simulink model "sample_system"  (R2022a)
settings: Solver=VariableStepAuto  StartTime=0  StopTime=t_sim_stop  RelTol=1e-3
values from neighbouring files (symbols this model uses):
  A = (pi/4)*(d_inj*.0254)^2    (= 1.14009182797e-05)    [Run_sim.m]
  attack_final_deviations = zeros(n_meas,1)    [Plot_attack_performance.m]    (also in Run_sim.m; find_non_trip_attack.m; get_simulation_object_sample_system.m; mymodelLoss.m)
  attack_full_times = attack_start_times +  100    [Plot_attack_performance.m]    (also in Run_sim.m = attack_start_times + 100; find_non_trip_attack.m; get_simulation_object_sample_system.m = attack_start_times +  10; mymodelLoss.m = attack_start_times +  10)
  attack_start_times = attack_start_injection*ones(n_meas,1)    [Plot_attack_performance.m]    (also in Run_sim.m; find_non_trip_attack.m; get_simulation_object_sample_system.m = 2*ones(n_meas,1); mymodelLoss.m = 2*ones(n_meas,1))
  Cd = 0.001    [Run_sim.m]
  detection_start = 100    [Run_sim.m]
  eta = 0.1    [Run_sim.m]
  Kd = 20    [Run_sim.m]
  Ki = 20    [Run_sim.m]
  Kp = 50    [Run_sim.m]
  noise_seed = 23341    [Run_sim.m]
  P_in = 101325    [Run_sim.m]
  P_middle = 1.68*P_in    (= 170226)    [Run_sim.m]
  P_out = 2*1.68*P_in    (= 340452)    [Run_sim.m]
  q_ref = 10    [Run_sim.m]
  x0 = [0;0]    [Run_sim.m]
libraries: slpidlib x2
settings Model: SimulationMode=rapid-accelerator  Creator=Abelb  LastModifiedBy=Abelb
settings DataIOCC: SaveFormat=StructureWithTime
settings OptimizationCC: BlockReduction=off  BufferReuse=off
settings DebuggingCC: AlgebraicLoopMsg=none
settings HardwareCC: TargetBitPerPointer=64  TargetBitPerSizeT=64  TargetBitPerPtrDiffT=64  TargetLongLongMode=on  TargetIntDivRoundTo=Zero  TargetEndianess=LittleEndian  TargetWordSize=64  TargetHWDeviceType=MATLAB Host  ProdEqTarget=off
settings RTWCC: Description=Rapid Simulation Target  SystemTargetFile=rsim.tlc  TemplateMakefile=rsim_default_tmf  DLArmComputeVersion=19.05
settings RSimTargetCC: TargetLangStandard=C99 (ISO)  OptimizeReductions=off
settings ExplorerConfigSet: SimMechanicsOpenEditorOnUpdate=off

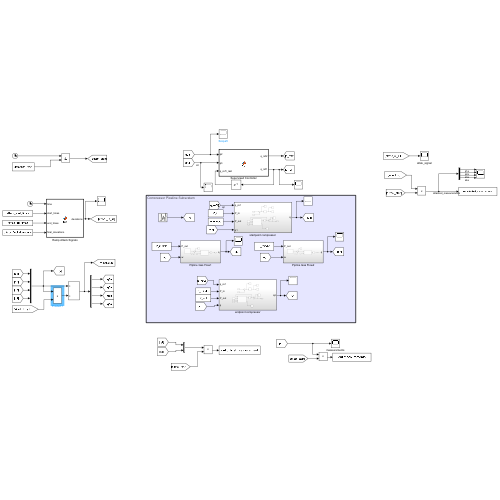
[thumbnail: Simulink's stored preview of the top-level diagram]
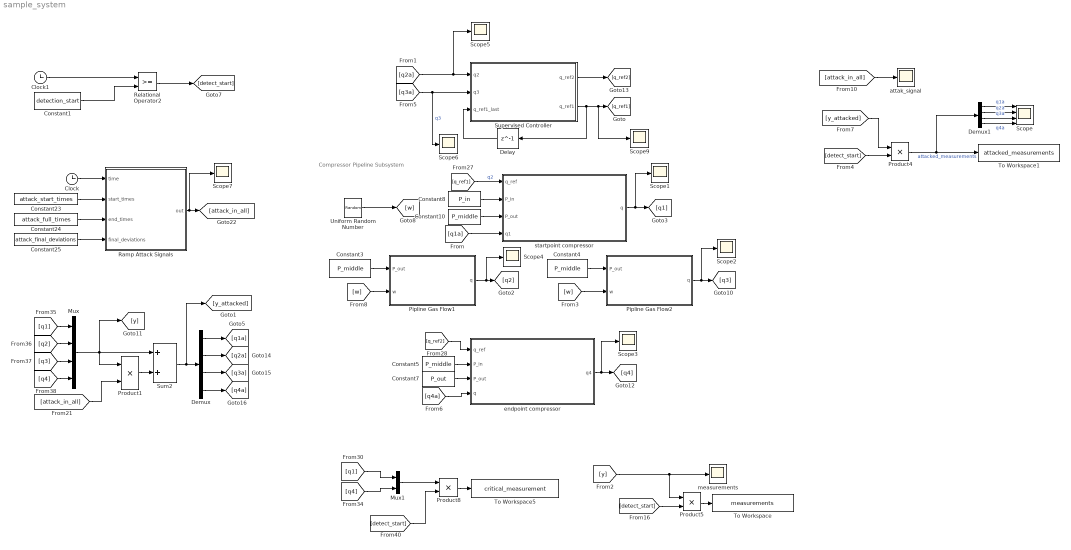
== system sample_system ==
  note: Compressor Pipeline Subsystem
  Clock : Clock
  Clock1 : Clock
  Constant1 : Constant  Value=detection_start
  Constant{3..5,10} (4 alike) : Constant  Value=P_middle
  Constant23 : Constant  Value=attack_start_times
  Constant24 : Constant  Value=attack_full_times
  Constant25 : Constant  Value=attack_final_deviations
  Constant7 : Constant  Value=P_out
  Constant8 : Constant  Value=P_in
  Delay : Delay  DelayLength=1
  Demux : Demux
  Demux1 : Demux
  Mux : Mux
  Mux1 : Mux  Inputs=2
  Pipline Gas Flow1 : Subsystem
  Pipline Gas Flow2 : Subsystem
  Product{1,4..5,8} (4 alike) : Product
  Ramp Attack Signals : MATLAB Function  TreatAsAtomicUnit=on
  Relational Operator2 : RelationalOperator  OutDataTypeStr=boolean  RndMeth=Simplest  InputSameDT=off
  Scope : Scope  NumInputPorts=4
  Scope{1..7,9} (8 alike) : Scope
  Sum2 : Sum
  Supervised Controller : MATLAB Function  TreatAsAtomicUnit=on
  To Workspace : ToWorkspace  VariableName=measurements  SaveFormat=Timeseries  SampleTime=-1
  To Workspace1 : ToWorkspace  VariableName=attacked_measurements  SaveFormat=Timeseries  SampleTime=-1
  To Workspace5 : ToWorkspace  VariableName=critical_measurement  SaveFormat=Timeseries  SampleTime=-1
  Uniform Random Number : UniformRandomNumber  Minimum=-0.01*P_middle  Maximum=0.01*P_middle  Seed=noise_seed  SampleTime=0.01
  attak_signal : Scope
  endpoint compressor : Subsystem
  measurements : Scope
  startpoint compressor : Subsystem
  wires:
  Clock1/1 -> Relational Operator2/1
  [y] -> Product5/1, measurements/1
  Relational Operator2/1 -> [detect_start]
  Constant1/1 -> Relational Operator2/2
  Uniform Random Number/1 -> [w]
  [detect_start] -> Product5/2
  Product5/1 -> To Workspace/1
  Constant24/1 -> Ramp Attack Signals/3(end_times)
  Clock/1 -> Ramp Attack Signals/1(time)
  Constant25/1 -> Ramp Attack Signals/4(final_deviations)
  Ramp Attack Signals/1(out) -> Scope7/1, [attack_in_all]
  Constant23/1 -> Ramp Attack Signals/2(start_times)
  [attack_in_all] -> attak_signal/1
  [attack_in_all] -> Product1/2
  Mux/1 -> [y], Product1/1, Sum2/1
  Product1/1 -> Sum2/2
  Sum2/1 -> [y_attacked], Demux/1
  Constant3/1 -> Pipline Gas Flow1/1(P_out)
  Pipline Gas Flow1/1(q) -> Scope4/1, [q2]
  Constant4/1 -> Pipline Gas Flow2/1(P_out)
  Pipline Gas Flow2/1(q) -> Scope2/1, [q3]
  [q_ref2] -> endpoint compressor/1(q_ref)
  Constant5/1 -> endpoint compressor/2(P_in)
  Constant7/1 -> endpoint compressor/3(P_out)
  startpoint compressor/1(q) -> Scope1/1, [q1]
  Constant10/1 -> startpoint compressor/3(P_out)
  Constant8/1 -> startpoint compressor/2(P_in)
  [w] -> Pipline Gas Flow2/2(w)
  [w] -> Pipline Gas Flow1/2(w)
  [q3a] -> Scope6/1, Supervised Controller/2(q3)  "q3"
  [q_ref1] -> startpoint compressor/1(q_ref)  "q2"
  [q2a] -> Scope5/1, Supervised Controller/1(q2)
  Supervised Controller/2(q_ref1) -> Scope9/1, [q_ref1], Delay/1
  Supervised Controller/1(q_ref2) -> [q_ref2]
  Delay/1 -> Supervised Controller/3(q_ref1_last)
  [q1a] -> startpoint compressor/4(q1)
  endpoint compressor/1(q4) -> Scope3/1, [q4]
  [q4a] -> endpoint compressor/4(q)
  [q1] -> Mux/1
  [q2] -> Mux/2
  [q3] -> Mux/3
  [q4] -> Mux/4
  Demux/1 -> [q1a]
  Demux/2 -> [q2a]
  Demux/3 -> [q3a]
  Demux/4 -> [q4a]
  Mux1/1 -> Product8/1
  [q1] -> Mux1/1
  [q4] -> Mux1/2
  [detect_start] -> Product8/2
  Product8/1 -> To Workspace5/1
  [detect_start] -> Product4/2
  [y_attacked] -> Product4/1
  Product4/1 -> Demux1/1, To Workspace1/1  "attacked_measurements"
  Demux1/1 -> Scope/1  "q1a"
  Demux1/2 -> Scope/2  "q2a"
  Demux1/3 -> Scope/3  "q3a"
  Demux1/4 -> Scope/4  "q4a"

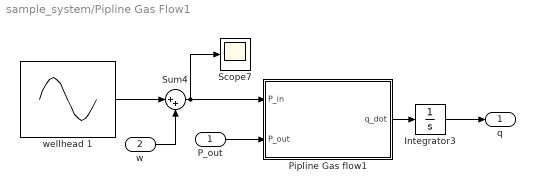
== system sample_system/Pipline Gas Flow1 ==
  P_out : Inport
  w : Inport  Port=2
  Integrator3 : Integrator
  Pipline Gas flow1 : MATLAB Function  TreatAsAtomicUnit=on
  Scope7 : Scope
  Sum4 : Sum  Inputs=|++
  wellhead 1 : Sin  Amplitude=0.1*P_middle  Bias=P_middle  Frequency=0.003  SampleTime=0
  q : Outport
  wires:
  Sum4/1 -> Scope7/1, Pipline Gas flow1/1(P_in)
  w/1 -> Sum4/2
  Pipline Gas flow1/1(q_dot) -> Integrator3/1
  Integrator3/1 -> q/1
  wellhead 1/1 -> Sum4/1
  P_out/1 -> Pipline Gas flow1/2(P_out)

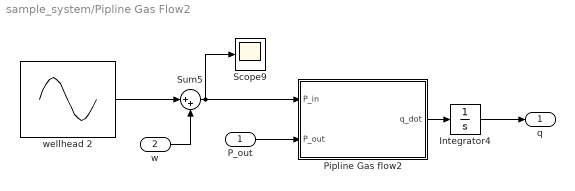
== system sample_system/Pipline Gas Flow2 ==
  P_out : Inport
  w : Inport  Port=2
  Integrator4 : Integrator
  Pipline Gas flow2 : MATLAB Function  TreatAsAtomicUnit=on
  Scope9 : Scope
  Sum5 : Sum  Inputs=|++
  wellhead 2 : Sin  Amplitude=0.1*P_middle  Bias=P_middle  Frequency=0.008  SampleTime=0
  q : Outport
  wires:
  Sum5/1 -> Scope9/1, Pipline Gas flow2/1(P_in)
  Pipline Gas flow2/1(q_dot) -> Integrator4/1
  Integrator4/1 -> q/1
  wellhead 2/1 -> Sum5/1
  w/1 -> Sum5/2
  P_out/1 -> Pipline Gas flow2/2(P_out)

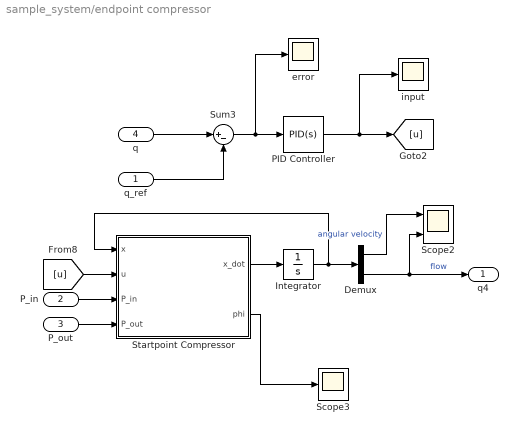
== system sample_system/endpoint compressor ==
  q_ref : Inport
  P_in : Inport  Port=2
  P_out : Inport  Port=3
  q : Inport  Port=4
  Demux : Demux  Outputs=2
  Integrator : Integrator  InitialCondition=x0
  PID Controller : slpidlib/PID Controller  Controller=PID  Form=Parallel  TimeDomain=Continuous-time  UseExternalTs=off  SampleTime=-1  IntegratorMethod=Forward Euler  FilterMethod=Forward Euler  ControllerParametersSource=internal  P=Kp  I=Ki  UseKiTs=off  D=Kd  N=100  UseFilter=on  TunerSelectOption=Transfer Function Based (PID Tuner App)  InitialConditionSource=internal  InitialConditionForIntegrator=0  InitialConditionForFilter=0  DifferentiatorICPrevScaledInput=0  ExternalReset=none  TrackingMode=off  Kt=1  LimitOutput=off  SatLimitsSource=internal  UpperSaturationLimit=inf  LowerSaturationLimit=-inf  LinearizeAsGain=on  AntiWindupMode=none  Kb=1  POutMin=[]  POutMax=[]  IOutMin=[]  IOutMax=[]  DOutMin=[]  DOutMax=[]  NOutMin=[]  NOutMax=[]  SumOutMin=[]  SumOutMax=[]  SaturationOutMin=[]  SaturationOutMax=[]  PParamMin=[]  PParamMax=[]  IParamMin=[]  IParamMax=[]  DParamMin=[]  DParamMax=[]  NParamMin=[]  NParamMax=[]  KbParamMin=[]  KbParamMax=[]  KtParamMin=[]  KtParamMax=[]  KbOutMin=[]  KbOutMax=[]  KtOutMin=[]  KtOutMax=[]  IntegratorOutMin=[]  IntegratorOutMax=[]  FilterOutMin=[]  FilterOutMax=[]  SumI1OutMin=[]  SumI1OutMax=[]  SumI2OutMin=[]  SumI2OutMax=[]  SumI3OutMin=[]  SumI3OutMax=[]  SumI4OutMin=[]  SumI4OutMax=[]  SumDOutMin=[]  SumDOutMax=[]  DifferentiatorOutMin=[]  DifferentiatorOutMax=[]  FilterDiffOutCoefMin=[]  FilterDiffOutCoefMax=[]  ReciprocalOutMin=[]  ReciprocalOutMax=[]  SumDenOutMin=[]  SumDenOutMax=[]  SumNumOutMin=[]  SumNumOutMax=[]  DivideOutMin=[]  DivideOutMax=[]  UdiffTsProdOutMin=[]  UdiffTsProdOutMax=[]  NTsProdOutMin=[]  NTsProdOutMax=[]  UintegralTsProdOutMin=[]  UintegralTsProdOutMax=[]  UngainTsProdOutMin=[]  UngainTsProdOutMax=[]  IntegratorContinuousStateAttributes=''  IntegratorStateMustResolveToSignalObject=off  IntegratorRTWStateStorageClass=Auto  FilterContinuousStateAttributes=''  FilterStateMustResolveToSignalObject=off  FilterRTWStateStorageClass=Auto  ParallelPVariant=InternalParameters  IdealPVariant=Disabled  IVariant=InternalParameters  DVariant=InternalParameters  IntegratorVariant=Continuous  SatVariant=Disabled  AWVariant=Passthrough  PCopyVariant=Disabled  TRVariant=Disabled  FdbkBlocksVariant=Forward  IdealPFdbkVariant=Disabled  SatFdbkVariant=Disabled  DerivativeFilterVariant=ContFilter  NVariant=InternalParameters  NCopyVariant=Disabled  FilterICVariant=InternalICsFilter  IntegratorICVariant=InternalICs  ExternalResetVariant=Disabled  TRSumVariant=Passthrough  SumFdbkVariant=Disabled  SumVariant=Sum_PID  TsampFilterVariant=InternalTs  TsampNgainVariant=Passthrough  TsampIntegralVariant=Passthrough  ExternalSaturationOutDataTypeStr=Inherit: Same as second input  aMode=0
  Scope2 : Scope  NumInputPorts=2
  Scope3 : Scope
  Startpoint Compressor : MATLAB Function  TreatAsAtomicUnit=on
  Sum3 : Sum  Inputs=|+-
  error : Scope
  input : Scope
  q4 : Outport
  wires:
  Demux/2 -> Scope2/2, q4/1  "flow"
  q/1 -> Sum3/1
  Demux/1 -> Scope2/1  "angular velocity"
  [u] -> Startpoint Compressor/2(u)
  Sum3/1 -> error/1, PID Controller/1
  q_ref/1 -> Sum3/2
  Startpoint Compressor/2(phi) -> Scope3/1
  Integrator/1 -> Startpoint Compressor/1(x), Demux/1
  Startpoint Compressor/1(x_dot) -> Integrator/1
  PID Controller/1 -> input/1, [u]
  P_in/1 -> Startpoint Compressor/3(P_in)
  P_out/1 -> Startpoint Compressor/4(P_out)

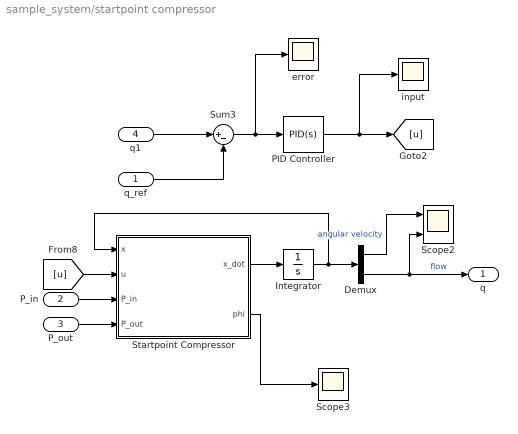
== system sample_system/startpoint compressor ==
  q_ref : Inport
  P_in : Inport  Port=2
  P_out : Inport  Port=3
  q1 : Inport  Port=4
  Demux : Demux  Outputs=2
  Integrator : Integrator  InitialCondition=x0
  PID Controller : slpidlib/PID Controller  Controller=PID  Form=Parallel  TimeDomain=Continuous-time  UseExternalTs=off  SampleTime=-1  IntegratorMethod=Forward Euler  FilterMethod=Forward Euler  ControllerParametersSource=internal  P=Kp  I=Ki  UseKiTs=off  D=Kd  N=100  UseFilter=on  TunerSelectOption=Transfer Function Based (PID Tuner App)  InitialConditionSource=internal  InitialConditionForIntegrator=0  InitialConditionForFilter=0  DifferentiatorICPrevScaledInput=0  ExternalReset=none  TrackingMode=off  Kt=1  LimitOutput=off  SatLimitsSource=internal  UpperSaturationLimit=inf  LowerSaturationLimit=-inf  LinearizeAsGain=on  AntiWindupMode=none  Kb=1  POutMin=[]  POutMax=[]  IOutMin=[]  IOutMax=[]  DOutMin=[]  DOutMax=[]  NOutMin=[]  NOutMax=[]  SumOutMin=[]  SumOutMax=[]  SaturationOutMin=[]  SaturationOutMax=[]  PParamMin=[]  PParamMax=[]  IParamMin=[]  IParamMax=[]  DParamMin=[]  DParamMax=[]  NParamMin=[]  NParamMax=[]  KbParamMin=[]  KbParamMax=[]  KtParamMin=[]  KtParamMax=[]  KbOutMin=[]  KbOutMax=[]  KtOutMin=[]  KtOutMax=[]  IntegratorOutMin=[]  IntegratorOutMax=[]  FilterOutMin=[]  FilterOutMax=[]  SumI1OutMin=[]  SumI1OutMax=[]  SumI2OutMin=[]  SumI2OutMax=[]  SumI3OutMin=[]  SumI3OutMax=[]  SumI4OutMin=[]  SumI4OutMax=[]  SumDOutMin=[]  SumDOutMax=[]  DifferentiatorOutMin=[]  DifferentiatorOutMax=[]  FilterDiffOutCoefMin=[]  FilterDiffOutCoefMax=[]  ReciprocalOutMin=[]  ReciprocalOutMax=[]  SumDenOutMin=[]  SumDenOutMax=[]  SumNumOutMin=[]  SumNumOutMax=[]  DivideOutMin=[]  DivideOutMax=[]  UdiffTsProdOutMin=[]  UdiffTsProdOutMax=[]  NTsProdOutMin=[]  NTsProdOutMax=[]  UintegralTsProdOutMin=[]  UintegralTsProdOutMax=[]  UngainTsProdOutMin=[]  UngainTsProdOutMax=[]  IntegratorContinuousStateAttributes=''  IntegratorStateMustResolveToSignalObject=off  IntegratorRTWStateStorageClass=Auto  FilterContinuousStateAttributes=''  FilterStateMustResolveToSignalObject=off  FilterRTWStateStorageClass=Auto  ParallelPVariant=InternalParameters  IdealPVariant=Disabled  IVariant=InternalParameters  DVariant=InternalParameters  IntegratorVariant=Continuous  SatVariant=Disabled  AWVariant=Passthrough  PCopyVariant=Disabled  TRVariant=Disabled  FdbkBlocksVariant=Forward  IdealPFdbkVariant=Disabled  SatFdbkVariant=Disabled  DerivativeFilterVariant=ContFilter  NVariant=InternalParameters  NCopyVariant=Disabled  FilterICVariant=InternalICsFilter  IntegratorICVariant=InternalICs  ExternalResetVariant=Disabled  TRSumVariant=Passthrough  SumFdbkVariant=Disabled  SumVariant=Sum_PID  TsampFilterVariant=InternalTs  TsampNgainVariant=Passthrough  TsampIntegralVariant=Passthrough  ExternalSaturationOutDataTypeStr=Inherit: Same as second input  aMode=0
  Scope2 : Scope  NumInputPorts=2
  Scope3 : Scope
  Startpoint Compressor : MATLAB Function  TreatAsAtomicUnit=on
  Sum3 : Sum  Inputs=|+-
  error : Scope
  input : Scope
  q : Outport
  wires:
  Demux/2 -> Scope2/2, q/1  "flow"
  Demux/1 -> Scope2/1  "angular velocity"
  [u] -> Startpoint Compressor/2(u)
  Sum3/1 -> error/1, PID Controller/1
  q_ref/1 -> Sum3/2
  Startpoint Compressor/2(phi) -> Scope3/1
  Integrator/1 -> Startpoint Compressor/1(x), Demux/1
  Startpoint Compressor/1(x_dot) -> Integrator/1
  PID Controller/1 -> input/1, [u]
  P_in/1 -> Startpoint Compressor/3(P_in)
  P_out/1 -> Startpoint Compressor/4(P_out)
  q1/1 -> Sum3/1

== matlab function sample_system/Supervised Controller ==
  data: q_ref2 output; q2 input; q3 input; q_ref1_last input; q_ref1 output; q_ref parameter; eta parameter
function [q_ref2,q_ref1]  = fcn(q2,q3,q_ref1_last,q_ref,eta)
%% Supervised control
% Minimize    1/2 * (q_ref1(k) - q_ref1(k-1))^2
% Subject to  |q_ref1(k) - q_ref| <= gamma*q_ref;
%             |q_ref1(k) + q2 - q_ref| <= gamma*q_ref;
%             |q_ref1(k) + q2 + q3 - q_ref| <= gamma*q_ref;
%
% Yu Zheng, Florida State University, 09/08/2022

upper_bound = (1+eta)*q_ref-q2-q3;
lower_bound = (1-eta)*q_ref;

if (q_ref1_last >= lower_bound) && (q_ref1_last <= upper_bound)
    q_ref1 = q_ref1_last;
elseif q_ref1_last < lower_bound
    q_ref1 = lower_bound;
else
    q_ref1 = upper_bound;
end

q_ref2 = q_ref1 + q2 + q3;

== matlab function sample_system/Ramp Attack Signals ==
  data: time input; out output; start_times input; end_times input; final_deviations input
function out = fcn(time,start_times,end_times,final_deviations)

delta_times = max(end_times-start_times,0);
ramp_rates  = final_deviations./delta_times;

deviations = (time<=start_times).*zeros(size(delta_times)) ...
    + ((time>start_times) & (time<=end_times)).*(ramp_rates.*(time-start_times)) ...
    + (time>end_times).*(final_deviations);

out = deviations.';

== matlab function sample_system/startpoint compressor/Startpoint Compressor ==
  data: x_dot output; x input; u input; param parameter; phi output; P_in input; P_out input
function [x_dot,phi]   = fcn(x,u,param, P_in, P_out)

%% unpack parameters and inputs
w = x(1);
q = x(2);

a   = param{1,1};
b   = param{1,2};
c1  = param{1,3};
c2  = param{1,4};
c12 = param{1,5};
c3  = param{1,6};
d   = param{1,7};


%% dynamical model
w_dot = a*u + b*q*w;
phi = (c1*w^2 + c2*q^2 + c12*w*q + c3)^6;
q_dot = d*(phi*P_in - P_out);


%% pack output
x_dot = [w_dot;
         q_dot];

== matlab function sample_system/endpoint compressor/Startpoint Compressor ==
  data: x_dot output; x input; u input; param parameter; phi output; P_in input; P_out input
function [x_dot,phi]   = fcn(x,u,param, P_in, P_out)

%% unpack parameters and inputs
w = x(1);
q = x(2);

a   = param{1,1};
b   = param{1,2};
c1  = param{1,3};
c2  = param{1,4};
c12 = param{1,5};
c3  = param{1,6};
d   = param{1,7};


%% dynamical model
w_dot = a*u + b*q*w;
phi = (c1*w^2 + c2*q^2 + c12*w*q + c3)^6;
q_dot = d*(phi*P_in - P_out);


%% pack output
x_dot = [w_dot;
         q_dot];

== matlab function sample_system/Pipline Gas Flow2/Pipline Gas flow2 ==
  data: P_in input; q_dot output; P_out input; A parameter; Cd parameter
function q_dot = fcn(P_in, P_out,A,Cd)

q_dot = A*Cd*(P_in - P_out);

== matlab function sample_system/Pipline Gas Flow1/Pipline Gas flow1 ==
  data: P_in input; q_dot output; P_out input; A parameter; Cd parameter
function q_dot = fcn(P_in, P_out,A,Cd)

q_dot = A*Cd*(P_in - P_out);
